simulink model "untitled"  (Simulink 9.1)
settings: Solver=VariableStepAuto  StartTime=0.0  StopTime=100  FixedStep=0.2  RelTol=1e-3
values from neighbouring files (symbols this model uses):
  A2 = A2G * A3 * A2D    [CCTR_Script_MoteurCourantContinu.m]    (also in CCTR_Script_MoteurCourantContinu_editd_v3.m; CCTR_Script_MoteurCourantContinubis.m)
  B2 = B2G * ( B3 + A3 * [beta; 0; 0])    [CCTR_Script_MoteurCourantContinu.m]    (also in CCTR_Script_MoteurCourantContinu_editd_v3.m; CCTR_Script_MoteurCourantContinubis.m)
  C2 = [ Kg  0 ... (first row only)    [CCTR_Script_MoteurCourantContinu.m]    (also in CCTR_Script_MoteurCourantContinu_editd_v3.m = [Kg 0;0 Ks*Kr ]; CCTR_Script_MoteurCourantContinubis.m = [ 1 1 ])
  G = acker(A2',C2(1,:)',poles_des)'    [CCTR_Script_MoteurCourantContinu_editd_v3.m]
  K = Ka(2:3)    [CCTR_Script_MoteurCourantContinu_editd_v3.m]
  Ka = acker(Aa, -Ba, poles_rt)    [CCTR_Script_MoteurCourantContinu.m]    (also in CCTR_Script_MoteurCourantContinu_editd_v3.m = acker(Aa,-Ba,poles_rt))
settings Model: Creator=Florian  LastModifiedBy=Florian
settings DataIOCC: SaveFormat=Dataset  ReturnWorkspaceOutputs=on
settings OptimizationCC: LifeSpan=auto
settings DebuggingCC: UnderspecifiedInitializationDetection=Simplified  MergeDetectMultiDrivingBlocksExec=error  UnconnectedInputMsg=none  UnconnectedOutputMsg=none  UnconnectedLineMsg=none  SFUnexpectedBacktrackingDiag=error  SFNoUnconditionalDefaultTransitionDiag=error  SFExecutionAtInitializationDiag=warning  SFMachineParentedDataDiag=error
settings HardwareCC: ProdBitPerPointer=64  ProdBitPerSizeT=64  ProdBitPerPtrDiffT=64  ProdLargestAtomicFloat=Float  ProdIntDivRoundTo=Zero  ProdEndianess=LittleEndian  ProdWordSize=64  ProdHWDeviceType=Intel->x86-64 (Windows64)
settings ModelReferenceCC: EnableRefExpFcnMdlSchedulingChecks=off  PropagateSignalLabelsOutOfModel=on
settings SFSimCC: SimUseLocalCustomCode=on
settings RTWCC: RTWUseLocalCustomCode=on
settings CodeAppCC: StateflowObjectComments=off
settings GRTTargetCC: TargetLangStandard=C99 (ISO)  CombineOutputUpdateFcns=on  GRTInterface=off
settings ConfigComp: CovMetricSettings=dwe  CovSaveCumulativeToWorkspaceVar=off  CovSaveSingleToWorkspaceVar=off  CovExternalEMLEnable=on

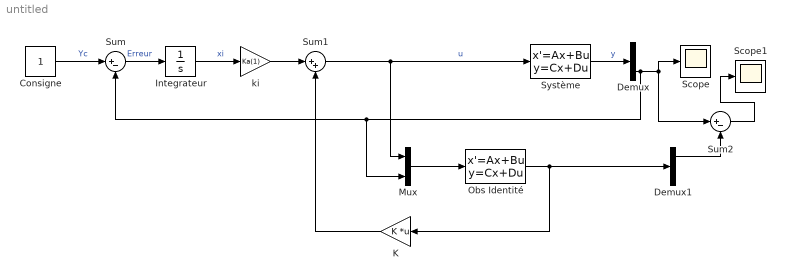
== system untitled ==
  Consigne : Constant
  Demux : Demux  Outputs=2
  Demux1 : Demux  Outputs=2
  Integrateur : Integrator
  K : Gain  Gain=K  Multiplication=Matrix(K*u)
  Mux : Mux  Inputs=2
  Obs Identité : StateSpace  A=A2-G*C2  B=[G B2]  C=eye(2)  D=[0 0; 0 0]  InitialCondition=[0 0]
  Scope : Scope
  Scope1 : Scope
  Sum : Sum  Inputs=|+-
  Sum1 : Sum  Inputs=|++
  Sum2 : Sum  Inputs=|+-
  Système : StateSpace  A=A2  B=B2  C=eye(2)  D=[0;0]  InitialCondition=0
  ki : Gain  Gain=Ka(1)
  wires:
  Consigne/1 -> Sum/1  "Yc"
  Sum/1 -> Integrateur/1  "Erreur"
  Integrateur/1 -> ki/1  "xi"
  ki/1 -> Sum1/1
  Sum1/1 -> Mux/1, Système/1  "u"
  Mux/1 -> Obs Identité/1
  Obs Identité/1 -> K/1, Demux1/1
  K/1 -> Sum1/2
  Système/1 -> Demux/1  "y"
  Sum2/1 -> Scope1/1
  Demux1/1 -> Sum2/2
  Demux/2 -> Sum/2, Mux/2, Sum2/1, Scope/1
